simulink model "trajectory_computation"  (R2021a)
settings: Solver=FixedStepAuto  StartTime=0.0  StopTime=inf  FixedStep=0.008  RelTol=1e-3
undefined symbols (not defined in the file): Tc
settings Model: Creator=Ruixuan  LastModifiedBy=Charles
settings SolverCC: ConcurrentTasks=on  PositivePriorityOrder=on  AutoInsertRateTranBlk=on  InsertRTBMode=Never (minimum delay)
settings DataIOCC: SaveOutput=off  SaveTime=off
settings OptimizationCC: BlockReduction=off  DefaultParameterBehavior=Inlined  OptimizeBlockIOStorage=off
settings DebuggingCC: TasksWithSamePriorityMsg=none
settings HardwareCC: ProdBitPerLong=64  ProdLongLongMode=on  ProdHWDeviceType=Intel->x86-64 (Linux 64)
settings ModelReferenceCC: ModelReferenceNumInstancesAllowed=Single
settings RTWCC: Description=Simulink Real-Time  SystemTargetFile=slrealtime.tlc  TemplateMakefile=slrealtime_default_tmf  Toolchain=Simulink Real-Time Toolchain  BuildConfiguration=Faster Runs  CodeExecutionProfiling=on  TargetLang=C++
settings SimulinkRealTimeTargetCC: ExtMode=off

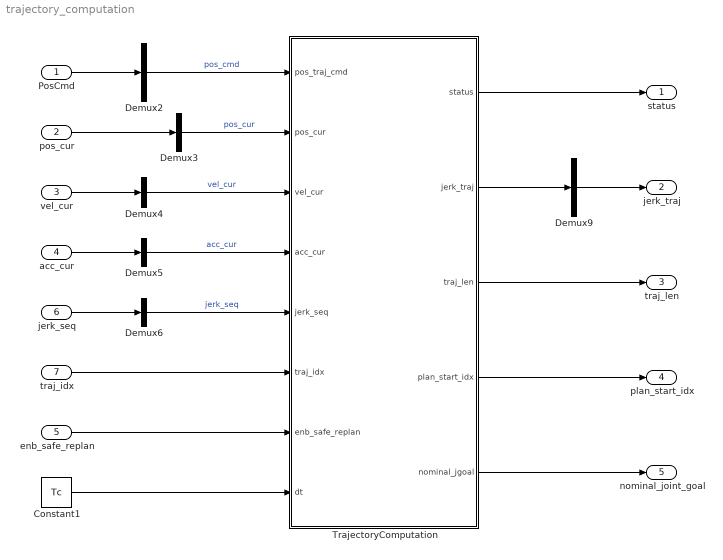
== system trajectory_computation ==
  PosCmd : Inport
  pos_cur : Inport  Port=2
  vel_cur : Inport  Port=3
  acc_cur : Inport  Port=4
  enb_safe_replan : Inport  Port=5
  jerk_seq : Inport  Port=6
  traj_idx : Inport  Port=7
  Constant1 : Constant  Value=Tc
  Demux2 : Demux  Outputs=[11255]
  Demux3 : Demux  Outputs=[6]
  Demux4 : Demux  Outputs=[6]
  Demux5 : Demux  Outputs=[6]
  Demux6 : Demux  Outputs=[30]
  Demux9 : Demux  Outputs=[11250]
  TrajectoryComputation : MATLAB Function  TreatAsAtomicUnit=on
  status : Outport  VectorParamsAs1DForOutWhenUnconnected=off
  jerk_traj : Outport  Port=2  VectorParamsAs1DForOutWhenUnconnected=off
  traj_len : Outport  Port=3  VectorParamsAs1DForOutWhenUnconnected=off
  plan_start_idx : Outport  Port=4  VectorParamsAs1DForOutWhenUnconnected=off
  nominal_joint_goal : Outport  Port=5  VectorParamsAs1DForOutWhenUnconnected=off
  wires:
  Constant1/1 -> TrajectoryComputation/8(dt)
  PosCmd/1 -> Demux2/1
  pos_cur/1 -> Demux3/1
  Demux2/1 -> TrajectoryComputation/1(pos_traj_cmd)  "pos_cmd"
  Demux3/1 -> TrajectoryComputation/2(pos_cur)  "pos_cur"
  traj_idx/1 -> TrajectoryComputation/6(traj_idx)
  TrajectoryComputation/1(status) -> status/1
  TrajectoryComputation/3(traj_len) -> traj_len/1
  TrajectoryComputation/4(plan_start_idx) -> plan_start_idx/1
  Demux4/1 -> TrajectoryComputation/3(vel_cur)  "vel_cur"
  vel_cur/1 -> Demux4/1
  Demux5/1 -> TrajectoryComputation/4(acc_cur)  "acc_cur"
  acc_cur/1 -> Demux5/1
  TrajectoryComputation/2(jerk_traj) -> Demux9/1
  Demux9/1 -> jerk_traj/1
  Demux6/1 -> TrajectoryComputation/5(jerk_seq)  "jerk_seq"
  jerk_seq/1 -> Demux6/1
  enb_safe_replan/1 -> TrajectoryComputation/7(enb_safe_replan)
  TrajectoryComputation/5(nominal_jgoal) -> nominal_joint_goal/1

== matlab function trajectory_computation/TrajectoryComputation ==
  data: status output; pos_traj_cmd input; pos_cur input; vel_cur input; acc_cur input; jerk_traj output; traj_len output; plan_start_idx output; jerk_seq input; traj_idx input; enb_safe_replan input; dt input; nominal_jgoal output
% This function computes the jerk-bounded nominal control command.
% Copyright (C) 2022  
% 
% Authors:
% Ruixuan Liu: ruixuanl@andrew.cmu.edu
% Rui Chen: ruic3@andrew.cmu.edu
% Changliu Liu : cliu6@andrew.cmu.edu
% 
% This program is free software; you can redistribute it and/or
% modify it under the terms of the GNU General Public License
% as published by the Free Software Foundation; either version 2
% of the License, or (at your option) any later version.
% 
% This program is distributed in the hope that it will be useful,
% but WITHOUT ANY WARRANTY; without even the implied warranty of
% MERCHANTABILITY or FITNESS FOR A PARTICULAR PURPOSE.  See the
% GNU General Public License for more details.
% 
% You should have received a copy of the GNU General Public License
% along with this program; if not, write to the Free Software
% Foundation, Inc., 51 Franklin Street, Fifth Floor, Boston, MA  02110-1301, USA.

function [status, jerk_traj, traj_len, plan_start_idx, nominal_jgoal] = TrajectoryComputation(pos_traj_cmd,pos_cur,vel_cur,acc_cur,... 
                                                                               jerk_seq,traj_idx,enb_safe_replan, dt)
    persistent m_seq m_goal;
    max_traj_len = 1875;

    % Initialize place holder.
    jerk_traj = zeros(max_traj_len*6, 1);
    nominal_jgoal = zeros(6,1);
    plan_start_idx = 0;
    traj_len = 0;
    if isempty(m_seq)
        m_seq = -1;
        m_goal = zeros(6, 1);
    end
    
    if ~enb_safe_replan
        % Command from host
        if pos_traj_cmd(end) == m_seq % No command.
            status = 0;
            nominal_jgoal(:) = m_goal(:);
            return;
        else
            m_seq = pos_traj_cmd(end);
        end
        leng = max(size(pos_traj_cmd, 2), size(pos_traj_cmd, 1));
        num_waypoints = pos_traj_cmd(leng - 4);
        override = min(max(pos_traj_cmd(leng - 1), 0.0001), 1);
        traj_hz = pos_traj_cmd(leng - 3);
        resample_hz = pos_traj_cmd(leng - 2);
        pos_cmd = pos_traj_cmd;
        if num_waypoints == 0
            num_waypoints = 1;
        end
        m_goal = pos_traj_cmd((num_waypoints-1)*6+1:(num_waypoints-1)*6+6);

    else
        % Command from internal SSA
        num_waypoints=1;
        override = 0.1;
        traj_hz = 0.25;
        resample_hz = 25;
        pos_cmd = pos_cur;%m_goal;%pos_cur;
    end
    nominal_jgoal(:) = m_goal(:);
    
    T = 1/traj_hz; % Traj freq
    K = resample_hz; % sampling freq
    K1 = T/dt/K;
    AdtK = A(dt*K1);
    BdtK = B(dt*K1);
    Adt = A(dt);
    Bdt = B(dt);
    pos_horizon = K*num_waypoints; % maximum task length
    
    if traj_idx ~=0
        % Has existing traj
        offset = 5;
        plan_start_idx = traj_idx + offset;
    else
        % Not existing traj
        plan_start_idx = 0;
    end
    
    pos_init = pos_cur;
    vel_init = vel_cur;
    acc_init = acc_cur;
    if enb_safe_replan
        pos_cmd = pos_init;
    end
    % Estimate future robot state
    for j=1:6
        for k=1:5
            x=[pos_init(j);vel_init(j);acc_init(j)];
            x=Adt*x + Bdt*jerk_seq((k-1)*6+j);
            pos_init(j) = x(1);
            vel_init(j) = x(2);
            acc_init(j) = x(3);
        end
    end
    
    for j = 1:6
        ref = zeros(num_waypoints + 2, 1);
        for i = 1:num_waypoints
            ref(i, 1) = pos_cmd(j+(i-1)*6);
        end
        pos = pos_init(j);
        vel = vel_init(j);
        acc = acc_init(j);
        xinit = [pos; vel; acc];
            
        uj = solveJerk(AdtK, BdtK, ref, xinit, num_waypoints, K);
        pos_T = 0;
        jerk_cnt = 0;
        traj_len = 0;
        
        for idx=1:max_traj_len
            pos_T = pos_T+1;
            if(mod(pos_T, floor(K1)) == 1 || floor(K1) == 1)
                jerk_cnt = jerk_cnt + 1;
                if(jerk_cnt > pos_horizon)
                    break;
                end
            end
            u = uj(jerk_cnt);
            jerk_traj(j+(idx-1)*6, 1) = u;
            traj_len = traj_len + 1;
        end
    end
   
    if 1/dt/K/traj_hz >= 1
        status = 1;
    else
        status = 0;
    end
    
    
function [Usol] = solveJerk(A, B, r, x0, N, K)
    xdim = size(A, 2);
    Abar = zeros(N+2, xdim);
    for i=1:K*N
        if(mod(i, K) == 0)
            Ai = A^i;
            cnt = i/K;
            if(cnt~=N)
                Abar(cnt, :) = Ai(1, :);
            else
                Abar(cnt:cnt+2, :) = Ai(:, :);
            end
        end
    end

    Bbar = zeros(N+2, N*K);
    for i=1:N*K
        if(mod(i, K) == 0)
            cnt = i/K;
            if(cnt~=N)
                idx = 1;
                nline = zeros(1, N*K);
                for j=(i-1):-1:0
                    AjB = A^j*B;
                    nline(:, idx) = AjB(1, :);
                    idx = idx + 1;
                end
                Bbar(cnt, :) = nline(1, :);
            else
                nline = zeros(xdim, N*K);
                idx = 1;
                for j=(i-1):-1:0
                    AjB = A^j*B;
                    nline(:, idx) = AjB;
                    idx = idx + 1;
                end
                Bbar(cnt:cnt+2, :) = nline;
            end
        end
    end

    Usol = Bbar\(r - Abar * x0);

function mtx = A(t)
    mtx = [1 t 0.5*t^2;
           0 1 t;
           0 0 1];
       
function mtx=B(t)
    mtx = [3/2*t^3; 0.5*t^2; t];
